simulink model "topology2"  (R2013a)
settings: Solver=ode4  StartTime=0.0  StopTime=0.5  FixedStep=1e-5  RelTol=1e-3
values from neighbouring files (symbols this model uses):
  Lload = Xload/wout_fund    [acemp_sixth.m]    (also in immd_base_varyingmod.m = Xload/wout; immd_design_elen.m = Xload/wout; immd_efficiency.m = Xload/wout; immd_simulation_base.m = Xload/wout)
  ma = 1    [IMMD_design_tool_v01.m]    (also in IMMD_design_tool_v02.m = 0.9; immd_base_varyingmod.m; immd_design_elen.m = 0.8; immd_efficiency.m = 0.85)
  phase = zeros(1,max_number_module)    [immd_base_varyingmod.m]    (also in immd_design_elen.m = [0 0 0 0]; immd_simulation_base.m = zeros(1,n))
  Rload = Zload*pf    [acemp_sixth.m]    (also in immd_base_varyingmod.m; immd_design_elen.m; immd_efficiency.m; immd_simulation_base.m)
  Ts = 1e-6    (= 1e-06)    [acemp_sixth.m]    (also in immd_base_varyingmod.m = 1e-05; immd_design_elen.m; immd_efficiency.m; immd_simulation_base.m = 1e-05)
  Vdc = (3/pi)*Vs_ll*sqrt(2)    [IMMD_design_tool_v01.m]    (also in IMMD_design_tool_v02.m; acemp_sixth.m = 400; immd_base_varyingmod.m = 400; immd_capacitor_rms_current.m = 400)
  wout = 2*pi*fout    (= 314.159265359)    [immd_base_varyingmod.m]    (also in immd_design_elen.m; immd_efficiency.m; immd_simulation_base.m)
libraries: powerlib x50, powerlib_meascontrol x24
settings Model: Creator=ugurm  LastModifiedBy=ugurm

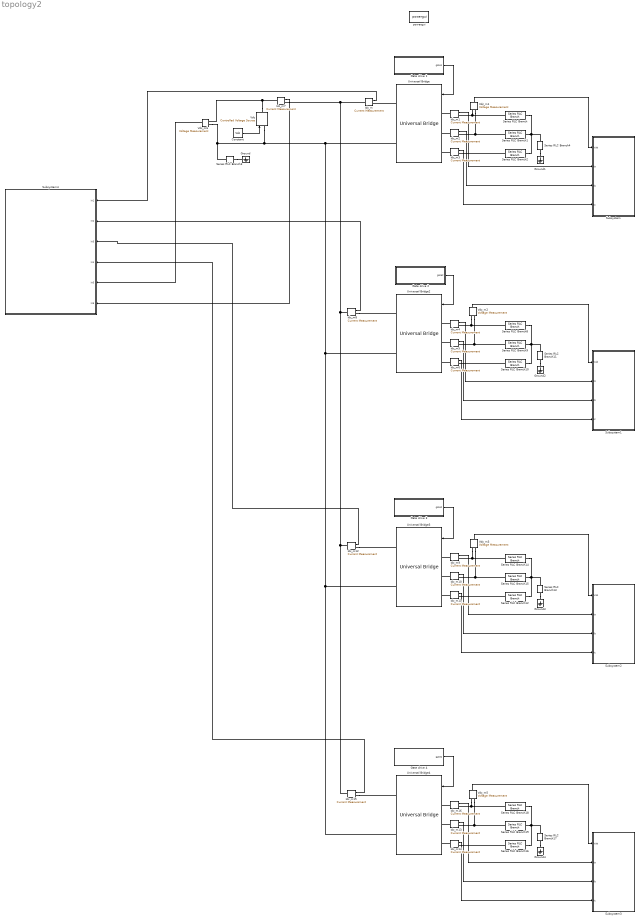
== system topology2 ==
  Constant : Constant  Value=Vdc
  Gate drive 1 : Subsystem
  Gate drive 2 : Subsystem
  Gate drive 3 : Subsystem
  Gate drive 4 : Subsystem
  Ground{,1..4} (5 alike) : powerlib/Elements/Ground  LConnTagsString=a
  Idc_m{,1..16} (17 alike) : powerlib/Measurements/Current Measurement  PhasorSimulation=off  OutputType=Complex  PSBequivalent=0
  Series RLC Branch{,1..2,8..10,12,14..16,18..19} (12 alike) : powerlib/Elements/Series RLC Branch  LConnTagsString=__new0  RConnTagsString=__new0  BranchType=RL  Resistance=Rload  Inductance=Lload  SetiL0=off  InitialCurrent=0  Capacitance=1e-6  Setx0=off  InitialVoltage=0  Measurements=None
  Series RLC Branch{3..4,11,13,17} (5 alike) : powerlib/Elements/Series RLC Branch  LConnTagsString=__new0  RConnTagsString=__new0  BranchType=R  Resistance=1e12  Inductance=Lload  SetiL0=off  InitialCurrent=0  Capacitance=1e-6  Setx0=off  InitialVoltage=0  Measurements=None
  Subsystem : Subsystem
  Subsystem1 : Subsystem
  Subsystem2 : Subsystem
  Subsystem3 : Subsystem
  Subsystem4 : Subsystem
  Universal Bridge{,2..4} (4 alike) : powerlib/Power Electronics/Universal Bridge  Arms=3  SnubberResistance=1e5  SnubberCapacitance=inf  Device=IGBT / Diodes  Ron=1e-6  Lon=0  ForwardVoltages="[  0  0  ]"  ForwardVoltage=0  GTOparameters=[ 10e-6 , 20e-6 ]  IGBTparameters=[ 1e-6 , 2e-6 ]  Measurements=None  Measurements_2=None  converterType=Rectifier
  Vdc : powerlib/Electrical Sources/Controlled Voltage Source  Initialize=off  Source_Type=DC  Amplitude=200  Phase=0  Frequency=0  Measurements=None
  Vdc_m{1..3,5..6} (5 alike) : powerlib/Measurements/Voltage Measurement  PhasorSimulation=off  OutputType=Complex  PSBequivalent=0
  powergui : powerlib/powergui  Priority=1  SimulationMode=Discrete  SolverType=Tustin  SampleTime=1e-5  frequency=60  SPID=off  DisableSnubberDevices=off  DisableRonSwitches=off  DisableVfSwitches=off  SwTol=0  Interpol=off  DisplayEquations=off  frequencyindice=0  Pbase=100e6  ErrMax=1e-4  Iterations=50  UnitsV=kV  UnitsW=MW  FunctionMessages=off  echomessages=off  HookPort=off  EnableUseOfTLC=off  x0status=blocks  RestoreLinks=warning  ResistiveCurrentMeasurement=off  Frange=[0:2:500]  Ylog=off  Xlog=on  ShowGrid=off  save=off  variable=ZData  structure=idc  ZoomFFT=off  StartTime=0.1  cycles=20  DisplayStyle=5  fundamental=50  FreqAxis=off  MaxFrequency=20000  frequencyindicesteady=1  RmsSteady=1  display=off  Ts=0  methode=off
  wires:
  Gate drive 1/1(gate1) -> Universal Bridge/1
  Idc_m4/1 -> Subsystem1/2(Ia)
  Idc_m5/1 -> Subsystem1/3(Ib)
  Idc_m6/1 -> Subsystem1/4(Ic)
  Vdc_m2/1 -> Subsystem1/1(Vab)
  Gate drive 2/1(gate2) -> Universal Bridge2/1
  Idc_m9/1 -> Subsystem2/2(Ia)
  Idc_m10/1 -> Subsystem2/3(Ib)
  Idc_m11/1 -> Subsystem2/4(Ic)
  Vdc_m3/1 -> Subsystem2/1(Vab)
  Gate drive 3/1(gate2) -> Universal Bridge3/1
  Idc_m16/1 -> Subsystem3/2(Ia)
  Idc_m13/1 -> Subsystem3/3(Ib)
  Idc_m14/1 -> Subsystem3/4(Ic)
  Vdc_m5/1 -> Subsystem3/1(Vab)
  Gate drive 4/1(gate2) -> Universal Bridge4/1
  Vdc_m1/1 -> Subsystem/1(Vab)
  Idc_m1/1 -> Subsystem/2(Ia)
  Idc_m2/1 -> Subsystem/3(Ib)
  Idc_m3/1 -> Subsystem/4(Ic)
  Idc_m/1 -> Subsystem4/1(In1)
  Idc_m8/1 -> Subsystem4/2(In2)
  Idc_m12/1 -> Subsystem4/3(In3)
  Idc_m15/1 -> Subsystem4/4(In4)
  Constant/1 -> Vdc/1
  Vdc_m6/1 -> Subsystem4/5(In5)
  Idc_m7/1 -> Subsystem4/6(In6)
  connections:
  Universal Bridge/RConn1 -- Idc_m/RConn1
  Vdc/LConn1 -- Series RLC Branch3/LConn1 -- Vdc_m6/LConn2 -- Universal Bridge4/RConn2 -- Universal Bridge3/RConn2 -- Universal Bridge2/RConn2 -- Universal Bridge/RConn2
  Idc_m1/LConn1 -- Universal Bridge/LConn1
  Idc_m2/LConn1 -- Universal Bridge/LConn2
  Idc_m3/LConn1 -- Universal Bridge/LConn3
  Series RLC Branch2/LConn1 -- Idc_m3/RConn1
  Series RLC Branch1/LConn1 -- Idc_m2/RConn1 -- Vdc_m1/LConn2
  Series RLC Branch/LConn1 -- Idc_m1/RConn1 -- Vdc_m1/LConn1
  Series RLC Branch/RConn1 -- Series RLC Branch4/LConn1 -- Series RLC Branch2/RConn1 -- Series RLC Branch1/RConn1
  Series RLC Branch4/RConn1 -- Ground1/LConn1
  Idc_m8/LConn1 -- Idc_m15/LConn1 -- Idc_m12/LConn1 -- Idc_m/LConn1 -- Idc_m7/RConn1
  Idc_m5/RConn1 -- Series RLC Branch9/LConn1 -- Vdc_m2/LConn2
  Idc_m4/RConn1 -- Series RLC Branch8/LConn1 -- Vdc_m2/LConn1
  Series RLC Branch9/RConn1 -- Series RLC Branch8/RConn1 -- Series RLC Branch11/LConn1 -- Series RLC Branch10/RConn1
  Idc_m6/LConn1 -- Universal Bridge2/LConn3
  Idc_m4/LConn1 -- Universal Bridge2/LConn1
  Series RLC Branch11/RConn1 -- Ground2/LConn1
  Idc_m5/LConn1 -- Universal Bridge2/LConn2
  Series RLC Branch10/LConn1 -- Idc_m6/RConn1
  Idc_m8/RConn1 -- Universal Bridge2/RConn1
  Vdc_m3/LConn2 -- Idc_m10/RConn1 -- Series RLC Branch15/LConn1
  Vdc_m3/LConn1 -- Idc_m9/RConn1 -- Series RLC Branch14/LConn1
  Series RLC Branch15/RConn1 -- Series RLC Branch14/RConn1 -- Series RLC Branch13/LConn1 -- Series RLC Branch12/RConn1
  Series RLC Branch12/LConn1 -- Idc_m11/RConn1
  Idc_m9/LConn1 -- Universal Bridge3/LConn1
  Idc_m11/LConn1 -- Universal Bridge3/LConn3
  Idc_m10/LConn1 -- Universal Bridge3/LConn2
  Idc_m12/RConn1 -- Universal Bridge3/RConn1
  Series RLC Branch13/RConn1 -- Ground3/LConn1
  Idc_m13/RConn1 -- Series RLC Branch19/LConn1 -- Vdc_m5/LConn2
  Idc_m16/RConn1 -- Series RLC Branch18/LConn1 -- Vdc_m5/LConn1
  Series RLC Branch19/RConn1 -- Series RLC Branch18/RConn1 -- Series RLC Branch17/LConn1 -- Series RLC Branch16/RConn1
  Series RLC Branch16/LConn1 -- Idc_m14/RConn1
  Idc_m16/LConn1 -- Universal Bridge4/LConn1
  Series RLC Branch17/RConn1 -- Ground4/LConn1
  Idc_m14/LConn1 -- Universal Bridge4/LConn3
  Idc_m13/LConn1 -- Universal Bridge4/LConn2
  Idc_m15/RConn1 -- Universal Bridge4/RConn1
  Vdc/RConn1 -- Vdc_m6/LConn1 -- Idc_m7/LConn1
  Series RLC Branch3/RConn1 -- Ground/LConn1

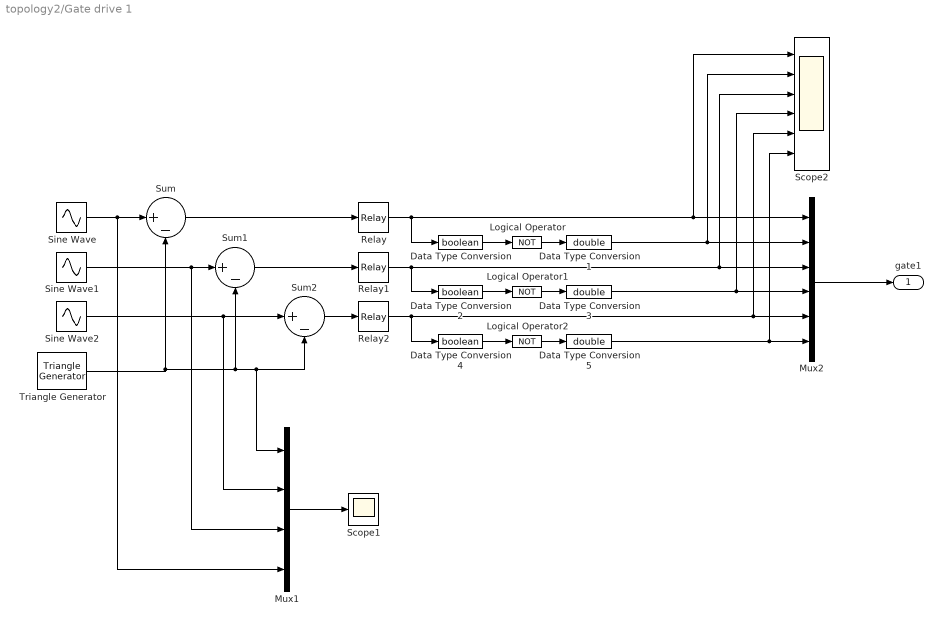
== system topology2/Gate drive 1 ==
  Data Type Conversion : DataTypeConversion  OutDataTypeStr=boolean
  Data Type Conversion1 : DataTypeConversion  OutDataTypeStr=double
  Data Type Conversion2 : DataTypeConversion  OutDataTypeStr=boolean
  Data Type Conversion3 : DataTypeConversion  OutDataTypeStr=double
  Data Type Conversion4 : DataTypeConversion  OutDataTypeStr=boolean
  Data Type Conversion5 : DataTypeConversion  OutDataTypeStr=double
  Logical Operator : Logic  Operator=NOT  AllPortsSameDT=off  OutDataTypeStr=boolean
  Logical Operator1 : Logic  Operator=NOT  AllPortsSameDT=off  OutDataTypeStr=boolean
  Logical Operator2 : Logic  Operator=NOT  AllPortsSameDT=off  OutDataTypeStr=boolean
  Mux1 : Mux
  Mux2 : Mux  Inputs=6
  Relay : Relay
  Relay1 : Relay
  Relay2 : Relay
  Scope1 : Scope
      settings: YMin=-1  YMax=1  SaveName=ScopeData4
  Scope2 : Scope  NumInputPorts=6
      settings: YMin=-2~-5~-5~-5~-5~-5  YMax=2~5~5~5~5~5  SaveName=ScopeData10
  Sine Wave : Sin  Amplitude=ma  Frequency=wout  SampleTime=0
  Sine Wave1 : Sin  Amplitude=ma  Frequency=wout  Phase=-2*pi/3  SampleTime=0
  Sine Wave2 : Sin  Amplitude=ma  Frequency=wout  Phase=2*pi/3  SampleTime=0
  Sum : Sum  Inputs=|+-
  Sum1 : Sum  Inputs=|+-
  Sum2 : Sum  Inputs=|+-
  Triangle Generator : powerlib_meascontrol/Pulse & Signal Generators/Triangle Generator  Freq=fsw  Phase=phase(1)  Ts=Ts
  gate1 : Outport
  wires:
  Sine Wave/1 -> Mux1/4, Sum/1
  Triangle Generator/1 -> Sum1/2, Mux1/1, Sum2/2, Sum/2
  Sine Wave1/1 -> Mux1/3, Sum1/1
  Sine Wave2/1 -> Mux1/2, Sum2/1
  Sum/1 -> Relay/1
  Sum1/1 -> Relay1/1
  Sum2/1 -> Relay2/1
  Data Type Conversion/1 -> Logical Operator/1
  Relay/1 -> Data Type Conversion/1, Scope2/1, Mux2/1
  Logical Operator/1 -> Data Type Conversion1/1
  Data Type Conversion1/1 -> Scope2/2, Mux2/2
  Data Type Conversion2/1 -> Logical Operator1/1
  Relay1/1 -> Data Type Conversion2/1, Scope2/3, Mux2/3
  Logical Operator1/1 -> Data Type Conversion3/1
  Data Type Conversion3/1 -> Scope2/4, Mux2/4
  Data Type Conversion4/1 -> Logical Operator2/1
  Relay2/1 -> Data Type Conversion4/1, Scope2/5, Mux2/5
  Logical Operator2/1 -> Data Type Conversion5/1
  Mux2/1 -> gate1/1
  Mux1/1 -> Scope1/1
  Data Type Conversion5/1 -> Scope2/6, Mux2/6

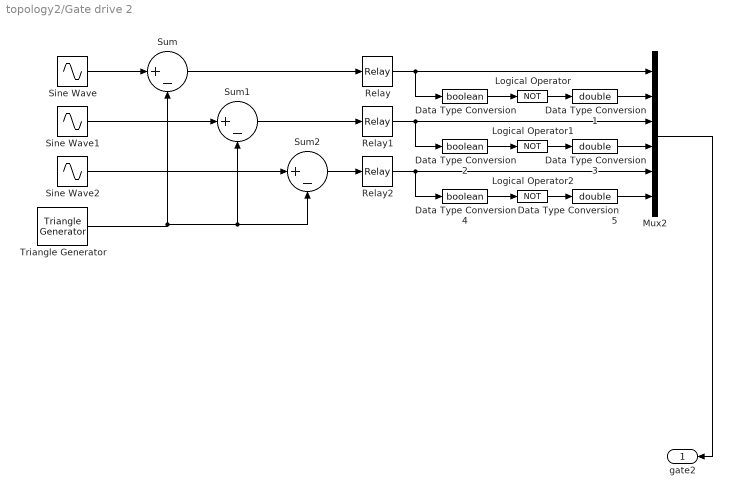
== system topology2/Gate drive 2 ==
  Data Type Conversion : DataTypeConversion  OutDataTypeStr=boolean
  Data Type Conversion1 : DataTypeConversion  OutDataTypeStr=double
  Data Type Conversion2 : DataTypeConversion  OutDataTypeStr=boolean
  Data Type Conversion3 : DataTypeConversion  OutDataTypeStr=double
  Data Type Conversion4 : DataTypeConversion  OutDataTypeStr=boolean
  Data Type Conversion5 : DataTypeConversion  OutDataTypeStr=double
  Logical Operator : Logic  Operator=NOT  AllPortsSameDT=off  OutDataTypeStr=boolean
  Logical Operator1 : Logic  Operator=NOT  AllPortsSameDT=off  OutDataTypeStr=boolean
  Logical Operator2 : Logic  Operator=NOT  AllPortsSameDT=off  OutDataTypeStr=boolean
  Mux2 : Mux  Inputs=6
  Relay : Relay
  Relay1 : Relay
  Relay2 : Relay
  Sine Wave : Sin  Amplitude=ma  Frequency=wout  SampleTime=0
  Sine Wave1 : Sin  Amplitude=ma  Frequency=wout  Phase=-2*pi/3  SampleTime=0
  Sine Wave2 : Sin  Amplitude=ma  Frequency=wout  Phase=2*pi/3  SampleTime=0
  Sum : Sum  Inputs=|+-
  Sum1 : Sum  Inputs=|+-
  Sum2 : Sum  Inputs=|+-
  Triangle Generator : powerlib_meascontrol/Pulse & Signal Generators/Triangle Generator  Freq=fsw  Phase=phase(2)  Ts=Ts
  gate2 : Outport
  wires:
  Sine Wave/1 -> Sum/1
  Triangle Generator/1 -> Sum1/2, Sum2/2, Sum/2
  Sine Wave1/1 -> Sum1/1
  Sine Wave2/1 -> Sum2/1
  Sum/1 -> Relay/1
  Sum1/1 -> Relay1/1
  Sum2/1 -> Relay2/1
  Data Type Conversion/1 -> Logical Operator/1
  Relay/1 -> Data Type Conversion/1, Mux2/1
  Logical Operator/1 -> Data Type Conversion1/1
  Data Type Conversion1/1 -> Mux2/2
  Data Type Conversion2/1 -> Logical Operator1/1
  Relay1/1 -> Data Type Conversion2/1, Mux2/3
  Logical Operator1/1 -> Data Type Conversion3/1
  Data Type Conversion3/1 -> Mux2/4
  Data Type Conversion4/1 -> Logical Operator2/1
  Relay2/1 -> Data Type Conversion4/1, Mux2/5
  Logical Operator2/1 -> Data Type Conversion5/1
  Data Type Conversion5/1 -> Mux2/6
  Mux2/1 -> gate2/1

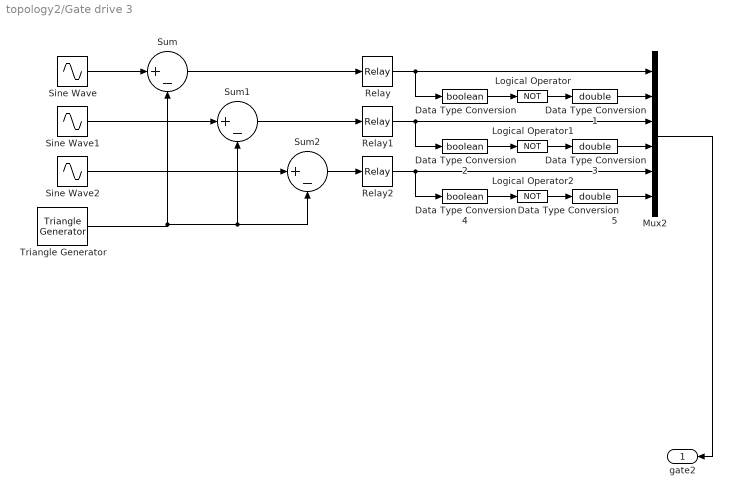
== system topology2/Gate drive 3 ==
  Data Type Conversion : DataTypeConversion  OutDataTypeStr=boolean
  Data Type Conversion1 : DataTypeConversion  OutDataTypeStr=double
  Data Type Conversion2 : DataTypeConversion  OutDataTypeStr=boolean
  Data Type Conversion3 : DataTypeConversion  OutDataTypeStr=double
  Data Type Conversion4 : DataTypeConversion  OutDataTypeStr=boolean
  Data Type Conversion5 : DataTypeConversion  OutDataTypeStr=double
  Logical Operator : Logic  Operator=NOT  AllPortsSameDT=off  OutDataTypeStr=boolean
  Logical Operator1 : Logic  Operator=NOT  AllPortsSameDT=off  OutDataTypeStr=boolean
  Logical Operator2 : Logic  Operator=NOT  AllPortsSameDT=off  OutDataTypeStr=boolean
  Mux2 : Mux  Inputs=6
  Relay : Relay
  Relay1 : Relay
  Relay2 : Relay
  Sine Wave : Sin  Amplitude=ma  Frequency=wout  SampleTime=0
  Sine Wave1 : Sin  Amplitude=ma  Frequency=wout  Phase=-2*pi/3  SampleTime=0
  Sine Wave2 : Sin  Amplitude=ma  Frequency=wout  Phase=2*pi/3  SampleTime=0
  Sum : Sum  Inputs=|+-
  Sum1 : Sum  Inputs=|+-
  Sum2 : Sum  Inputs=|+-
  Triangle Generator : powerlib_meascontrol/Pulse & Signal Generators/Triangle Generator  Freq=fsw  Phase=phase(3)  Ts=Ts
  gate2 : Outport
  wires:
  Sine Wave/1 -> Sum/1
  Triangle Generator/1 -> Sum1/2, Sum2/2, Sum/2
  Sine Wave1/1 -> Sum1/1
  Sine Wave2/1 -> Sum2/1
  Sum/1 -> Relay/1
  Sum1/1 -> Relay1/1
  Sum2/1 -> Relay2/1
  Data Type Conversion/1 -> Logical Operator/1
  Relay/1 -> Data Type Conversion/1, Mux2/1
  Logical Operator/1 -> Data Type Conversion1/1
  Data Type Conversion1/1 -> Mux2/2
  Data Type Conversion2/1 -> Logical Operator1/1
  Relay1/1 -> Data Type Conversion2/1, Mux2/3
  Logical Operator1/1 -> Data Type Conversion3/1
  Data Type Conversion3/1 -> Mux2/4
  Data Type Conversion4/1 -> Logical Operator2/1
  Relay2/1 -> Data Type Conversion4/1, Mux2/5
  Logical Operator2/1 -> Data Type Conversion5/1
  Data Type Conversion5/1 -> Mux2/6
  Mux2/1 -> gate2/1

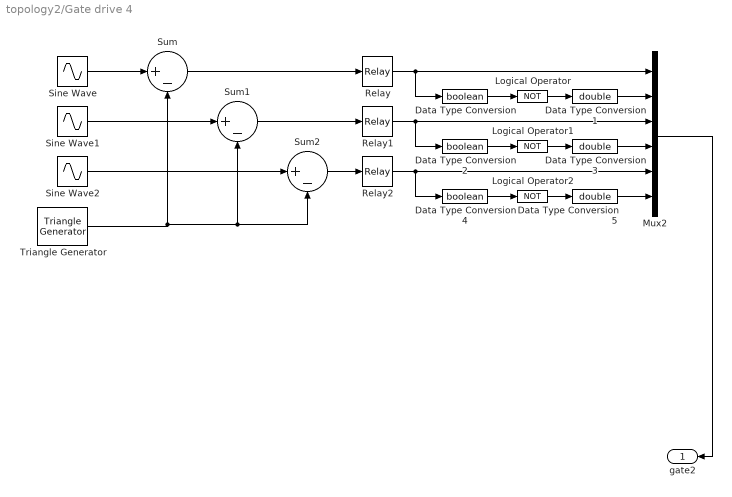
== system topology2/Gate drive 4 ==
  Data Type Conversion : DataTypeConversion  OutDataTypeStr=boolean
  Data Type Conversion1 : DataTypeConversion  OutDataTypeStr=double
  Data Type Conversion2 : DataTypeConversion  OutDataTypeStr=boolean
  Data Type Conversion3 : DataTypeConversion  OutDataTypeStr=double
  Data Type Conversion4 : DataTypeConversion  OutDataTypeStr=boolean
  Data Type Conversion5 : DataTypeConversion  OutDataTypeStr=double
  Logical Operator : Logic  Operator=NOT  AllPortsSameDT=off  OutDataTypeStr=boolean
  Logical Operator1 : Logic  Operator=NOT  AllPortsSameDT=off  OutDataTypeStr=boolean
  Logical Operator2 : Logic  Operator=NOT  AllPortsSameDT=off  OutDataTypeStr=boolean
  Mux2 : Mux  Inputs=6
  Relay : Relay
  Relay1 : Relay
  Relay2 : Relay
  Sine Wave : Sin  Amplitude=ma  Frequency=wout  SampleTime=0
  Sine Wave1 : Sin  Amplitude=ma  Frequency=wout  Phase=-2*pi/3  SampleTime=0
  Sine Wave2 : Sin  Amplitude=ma  Frequency=wout  Phase=2*pi/3  SampleTime=0
  Sum : Sum  Inputs=|+-
  Sum1 : Sum  Inputs=|+-
  Sum2 : Sum  Inputs=|+-
  Triangle Generator : powerlib_meascontrol/Pulse & Signal Generators/Triangle Generator  Freq=fsw  Phase=phase(4)  Ts=Ts
  gate2 : Outport
  wires:
  Sine Wave/1 -> Sum/1
  Triangle Generator/1 -> Sum1/2, Sum2/2, Sum/2
  Sine Wave1/1 -> Sum1/1
  Sine Wave2/1 -> Sum2/1
  Sum/1 -> Relay/1
  Sum1/1 -> Relay1/1
  Sum2/1 -> Relay2/1
  Data Type Conversion/1 -> Logical Operator/1
  Relay/1 -> Data Type Conversion/1, Mux2/1
  Logical Operator/1 -> Data Type Conversion1/1
  Data Type Conversion1/1 -> Mux2/2
  Data Type Conversion2/1 -> Logical Operator1/1
  Relay1/1 -> Data Type Conversion2/1, Mux2/3
  Logical Operator1/1 -> Data Type Conversion3/1
  Data Type Conversion3/1 -> Mux2/4
  Data Type Conversion4/1 -> Logical Operator2/1
  Relay2/1 -> Data Type Conversion4/1, Mux2/5
  Logical Operator2/1 -> Data Type Conversion5/1
  Data Type Conversion5/1 -> Mux2/6
  Mux2/1 -> gate2/1

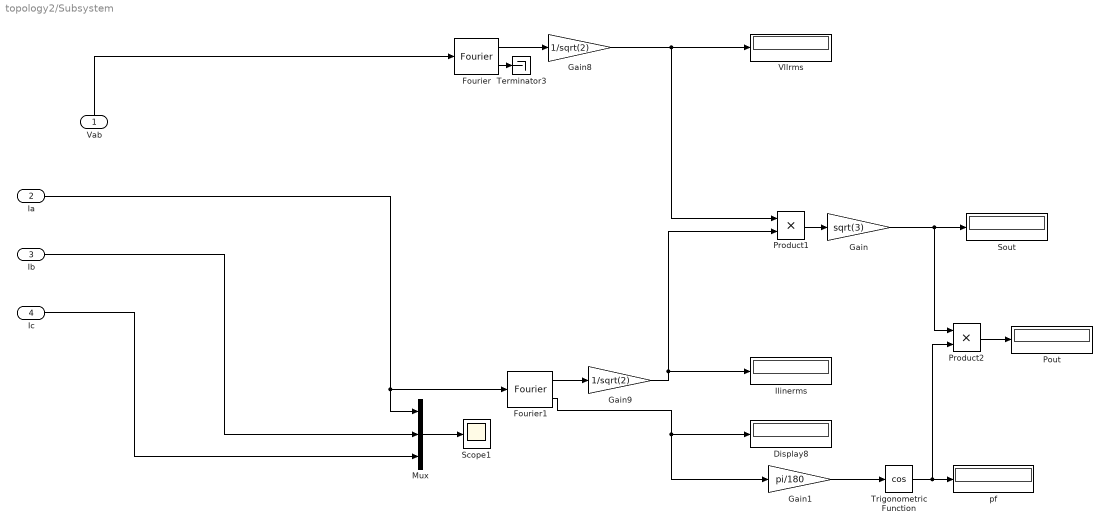
== system topology2/Subsystem ==
  Vab : Inport
  Ia : Inport  Port=2
  Ib : Inport  Port=3
  Ic : Inport  Port=4
  Display8 : Display
  Fourier : powerlib_meascontrol/Measurements/Fourier  Freq=fout  n=1  InInit=[0, 0]  Ts=0
  Fourier1 : powerlib_meascontrol/Measurements/Fourier  Freq=fout  n=1  InInit=[0, 0]  Ts=0
  Gain : Gain  Gain=sqrt(3)
  Gain1 : Gain  Gain=pi/180
  Gain8 : Gain  Gain=1/sqrt(2)
  Gain9 : Gain  Gain=1/sqrt(2)
  "Ilinerms " : Display
  Mux : Mux  Inputs=3
  Pout : Display
  Product1 : Product
  Product2 : Product
  Scope1 : Scope
      settings: YMin=-800  YMax=800
  Sout : Display
      settings: Format=short_e
  Terminator3 : Terminator
  Trigonometric Function : Trigonometry  Operator=cos
  "Vllrms " : Display
  pf : Display
  wires:
  Gain8/1 -> Product1/1, "Vllrms "/1
  Gain9/1 -> "Ilinerms "/1, Product1/2
  Ia/1 -> Mux/1, Fourier1/1
  Ib/1 -> Mux/2
  Ic/1 -> Mux/3
  Mux/1 -> Scope1/1
  Fourier1/1 -> Gain9/1
  Vab/1 -> Fourier/1
  Fourier/1 -> Gain8/1
  Product1/1 -> Gain/1
  Gain/1 -> Product2/1, Sout/1
  Fourier1/2 -> Gain1/1, Display8/1
  Trigonometric Function/1 -> Product2/2, pf/1
  Gain1/1 -> Trigonometric Function/1
  Product2/1 -> Pout/1
  Fourier/2 -> Terminator3/1

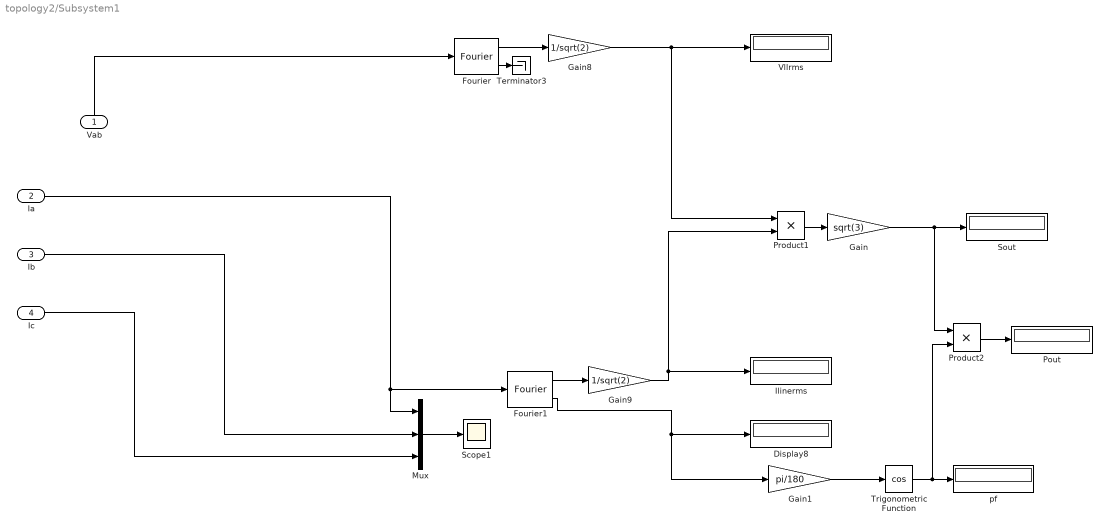
== system topology2/Subsystem1 ==
  Vab : Inport
  Ia : Inport  Port=2
  Ib : Inport  Port=3
  Ic : Inport  Port=4
  Display8 : Display
  Fourier : powerlib_meascontrol/Measurements/Fourier  Freq=fout  n=1  InInit=[0, 0]  Ts=0
  Fourier1 : powerlib_meascontrol/Measurements/Fourier  Freq=fout  n=1  InInit=[0, 0]  Ts=0
  Gain : Gain  Gain=sqrt(3)
  Gain1 : Gain  Gain=pi/180
  Gain8 : Gain  Gain=1/sqrt(2)
  Gain9 : Gain  Gain=1/sqrt(2)
  "Ilinerms " : Display
  Mux : Mux  Inputs=3
  Pout : Display
  Product1 : Product
  Product2 : Product
  Scope1 : Scope
      settings: YMin=500  YMax=800
  Sout : Display
      settings: Format=short_e
  Terminator3 : Terminator
  Trigonometric Function : Trigonometry  Operator=cos
  "Vllrms " : Display
  pf : Display
  wires:
  Gain8/1 -> Product1/1, "Vllrms "/1
  Gain9/1 -> "Ilinerms "/1, Product1/2
  Ia/1 -> Mux/1, Fourier1/1
  Ib/1 -> Mux/2
  Ic/1 -> Mux/3
  Mux/1 -> Scope1/1
  Fourier1/1 -> Gain9/1
  Vab/1 -> Fourier/1
  Fourier/1 -> Gain8/1
  Product1/1 -> Gain/1
  Gain/1 -> Product2/1, Sout/1
  Fourier1/2 -> Gain1/1, Display8/1
  Trigonometric Function/1 -> Product2/2, pf/1
  Gain1/1 -> Trigonometric Function/1
  Product2/1 -> Pout/1
  Fourier/2 -> Terminator3/1

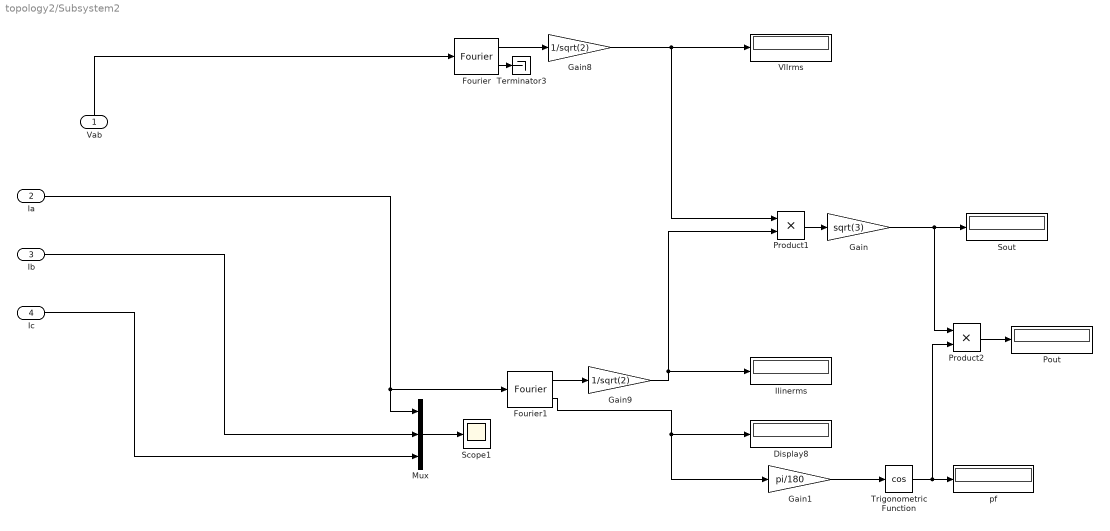
== system topology2/Subsystem2 ==
  Vab : Inport
  Ia : Inport  Port=2
  Ib : Inport  Port=3
  Ic : Inport  Port=4
  Display8 : Display
  Fourier : powerlib_meascontrol/Measurements/Fourier  Freq=fout  n=1  InInit=[0, 0]  Ts=0
  Fourier1 : powerlib_meascontrol/Measurements/Fourier  Freq=fout  n=1  InInit=[0, 0]  Ts=0
  Gain : Gain  Gain=sqrt(3)
  Gain1 : Gain  Gain=pi/180
  Gain8 : Gain  Gain=1/sqrt(2)
  Gain9 : Gain  Gain=1/sqrt(2)
  "Ilinerms " : Display
  Mux : Mux  Inputs=3
  Pout : Display
  Product1 : Product
  Product2 : Product
  Scope1 : Scope
      settings: YMin=500  YMax=800
  Sout : Display
      settings: Format=short_e
  Terminator3 : Terminator
  Trigonometric Function : Trigonometry  Operator=cos
  "Vllrms " : Display
  pf : Display
  wires:
  Gain8/1 -> Product1/1, "Vllrms "/1
  Gain9/1 -> "Ilinerms "/1, Product1/2
  Ia/1 -> Mux/1, Fourier1/1
  Ib/1 -> Mux/2
  Ic/1 -> Mux/3
  Mux/1 -> Scope1/1
  Fourier1/1 -> Gain9/1
  Vab/1 -> Fourier/1
  Fourier/1 -> Gain8/1
  Product1/1 -> Gain/1
  Gain/1 -> Product2/1, Sout/1
  Fourier1/2 -> Gain1/1, Display8/1
  Trigonometric Function/1 -> Product2/2, pf/1
  Gain1/1 -> Trigonometric Function/1
  Product2/1 -> Pout/1
  Fourier/2 -> Terminator3/1

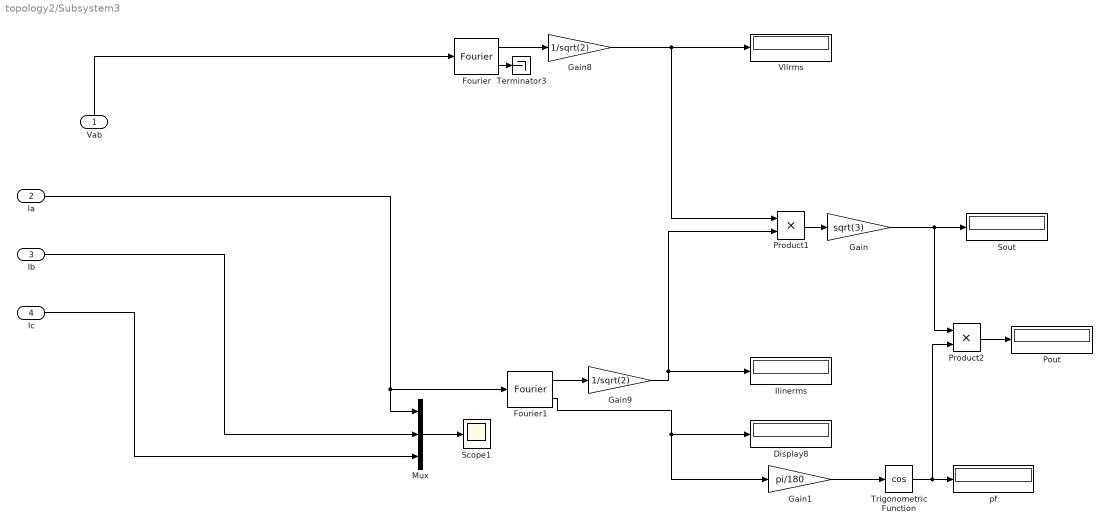
== system topology2/Subsystem3 ==
  Vab : Inport
  Ia : Inport  Port=2
  Ib : Inport  Port=3
  Ic : Inport  Port=4
  Display8 : Display
  Fourier : powerlib_meascontrol/Measurements/Fourier  Freq=fout  n=1  InInit=[0, 0]  Ts=0
  Fourier1 : powerlib_meascontrol/Measurements/Fourier  Freq=fout  n=1  InInit=[0, 0]  Ts=0
  Gain : Gain  Gain=sqrt(3)
  Gain1 : Gain  Gain=pi/180
  Gain8 : Gain  Gain=1/sqrt(2)
  Gain9 : Gain  Gain=1/sqrt(2)
  "Ilinerms " : Display
  Mux : Mux  Inputs=3
  Pout : Display
  Product1 : Product
  Product2 : Product
  Scope1 : Scope
      settings: YMin=500  YMax=800
  Sout : Display
      settings: Format=short_e
  Terminator3 : Terminator
  Trigonometric Function : Trigonometry  Operator=cos
  "Vllrms " : Display
  pf : Display
  wires:
  Gain8/1 -> Product1/1, "Vllrms "/1
  Gain9/1 -> "Ilinerms "/1, Product1/2
  Ia/1 -> Mux/1, Fourier1/1
  Ib/1 -> Mux/2
  Ic/1 -> Mux/3
  Mux/1 -> Scope1/1
  Fourier1/1 -> Gain9/1
  Vab/1 -> Fourier/1
  Fourier/1 -> Gain8/1
  Product1/1 -> Gain/1
  Gain/1 -> Product2/1, Sout/1
  Fourier1/2 -> Gain1/1, Display8/1
  Trigonometric Function/1 -> Product2/2, pf/1
  Gain1/1 -> Trigonometric Function/1
  Product2/1 -> Pout/1
  Fourier/2 -> Terminator3/1

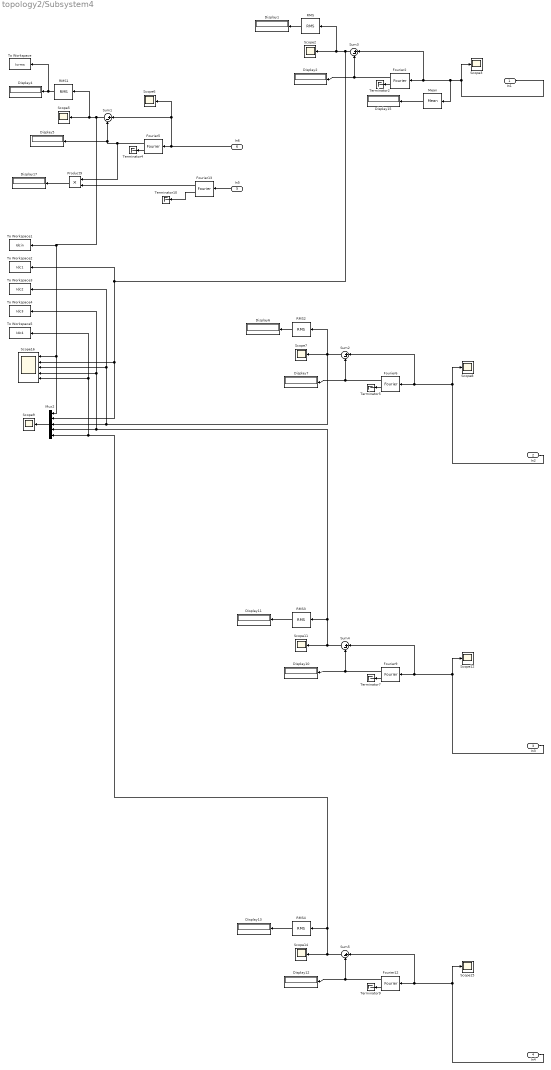
== system topology2/Subsystem4 ==
  In1 : Inport
  In2 : Inport  Port=2
  In3 : Inport  Port=3
  In4 : Inport  Port=4
  In5 : Inport  Port=5
  In6 : Inport  Port=6
  Display{1..2,4..7,10..13,15,17} (12 alike) : Display
  Fourier{2,5..6,9,12..13} (6 alike) : powerlib_meascontrol/Measurements/Fourier  Freq=fout  n=0  InInit=[0, 0]  Ts=0
  Mean : powerlib_meascontrol/Measurements/Mean  Freq=50  Vinit=0  Ts=0
  Mux2 : Mux  Inputs=5
  Product9 : Product
  RMS{,1..4} (5 alike) : powerlib_meascontrol/Measurements/RMS  TrueRMS=on  Freq=50  RMSInit=120  Ts=0
  Scope{2..3,5..9,11..12,14..15} (11 alike) : Scope
      Scope11 settings: YMin=-1.25  YMax=1.25  SaveName=ScopeData11
      Scope12 settings: YMin=500  YMax=800  SaveName=ScopeData12
      Scope14 settings: YMin=-1.25  YMax=1.25  SaveName=ScopeData14
      Scope15 settings: YMin=500  YMax=800  SaveName=ScopeData15
      Scope2 settings: YMin=-1.25  YMax=1.25  SaveName=ScopeData2
      Scope3 settings: YMin=-10  YMax=10  SaveName=ScopeData3
      Scope5 settings: YMin=-2.25e+63  YMax=2.5e+62  SaveName=ScopeData5
      Scope6 settings: YMin=500  YMax=800  SaveName=ScopeData6
      Scope7 settings: YMin=-1.25  YMax=1.25  SaveName=ScopeData7
      Scope8 settings: YMin=500  YMax=800  SaveName=ScopeData8
      Scope9 settings: YMin=-2.5  YMax=2  SaveName=ScopeData9
  Scope16 : Scope  NumInputPorts=5
      settings: YMin=-2.5~-5~-5~-5~-5  YMax=2~5~5~5~5  SaveName=Icaps
  Sum{1..5} (5 alike) : Sum  Inputs=|+-
  Terminator{2,4..5,7,9..10} (6 alike) : Terminator
  To Workspace : ToWorkspace  VariableName=Icrms  SampleTime=-1
  To Workspace1 : ToWorkspace  VariableName=Idcin  SampleTime=-1
  To Workspace2 : ToWorkspace  VariableName=Idc1  SampleTime=-1
  To Workspace3 : ToWorkspace  VariableName=Idc2  SampleTime=-1
  To Workspace4 : ToWorkspace  VariableName=Idc3  SampleTime=-1
  To Workspace5 : ToWorkspace  VariableName=Idc4  SampleTime=-1
  wires:
  Fourier13/2 -> Terminator10/1
  Fourier13/1 -> Product9/2
  Product9/1 -> Display17/1
  In4/1 -> Scope15/1, Sum5/1, Fourier12/1
  Fourier12/1 -> Sum5/2, Display12/1
  Fourier12/2 -> Terminator9/1
  Sum5/1 -> To Workspace5/1, Scope16/5, Mux2/5, RMS4/1, Scope14/1
  RMS4/1 -> Display13/1
  Mux2/1 -> Scope9/1
  RMS/1 -> Display1/1
  Mean/1 -> Display15/1
  RMS3/1 -> Display11/1
  Fourier9/1 -> Sum4/2, Display10/1
  In3/1 -> Scope12/1, Sum4/1, Fourier9/1
  Fourier9/2 -> Terminator7/1
  In6/1 -> Scope6/1, Sum1/1, Fourier5/1
  Fourier5/2 -> Terminator4/1
  RMS1/1 -> To Workspace/1, Display4/1
  Fourier5/1 -> Product9/1, Sum1/2, Display5/1
  Sum1/1 -> Scope16/1, Mux2/1, To Workspace1/1, RMS1/1, Scope5/1
  Sum3/1 -> Scope16/2, Mux2/2, To Workspace2/1, RMS/1, Scope2/1
  Fourier6/1 -> Sum2/2, Display7/1
  RMS2/1 -> Display6/1
  Fourier6/2 -> Terminator5/1
  In2/1 -> Scope8/1, Sum2/1, Fourier6/1
  In1/1 -> Scope3/1, Mean/1, Sum3/1, Fourier2/1
  Fourier2/1 -> Sum3/2, Display2/1
  Fourier2/2 -> Terminator2/1
  Sum2/1 -> RMS2/1, Scope16/3, To Workspace3/1, Mux2/3, Scope7/1
  Sum4/1 -> To Workspace4/1, Scope16/4, Mux2/4, RMS3/1, Scope11/1
  In5/1 -> Fourier13/1
